simulink library "cocosimLibs"  (R2017b)
settings: Solver=VariableStepAuto  StartTime=0.0  StopTime=10.0  RelTol=1e-3
settings Model: Creator=hbourbou  LastModifiedBy=hbourbou

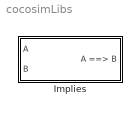
== system cocosimLibs ==
  Implies : Subsystem  TreatAsAtomicUnit=on

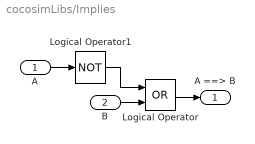
== system cocosimLibs/Implies ==
  A : Inport
  B : Inport  Port=2
  Logical Operator : Logic  Operator=OR  AllPortsSameDT=off  OutDataTypeStr=boolean
  Logical Operator1 : Logic  Operator=NOT  AllPortsSameDT=off  OutDataTypeStr=boolean
  A ==> B : Outport
  wires:
  Logical Operator1/1 -> Logical Operator/1
  Logical Operator/1 -> A ==> B/1
  A/1 -> Logical Operator1/1
  B/1 -> Logical Operator/2
